simulink model "mimo_sim1"  (R2014a)
settings: Solver=ode45  StartTime=0.0  StopTime=20  RelTol=1e-3
values from neighbouring files (symbols this model uses):
  A = [A_lat, B_lat; zeros(2,5), [A_da 0; 0 A_dr]]    [session3.m]
  B = [zeros(5,2); B_da 0; 0 B_dr]    [session3.m]
  C = eye(7)    [session3.m]
  D = zeros(7,2)    [session3.m]
  k_phi = 0.1    [session3.m]
  k_psi = 2    [session3.m]
  k_r = 0.002    [session3.m]
settings Model: Creator=Bella Kim  LastModifiedBy=Bella Kim
settings DebuggingCC: SolverPrmCheckMsg=none

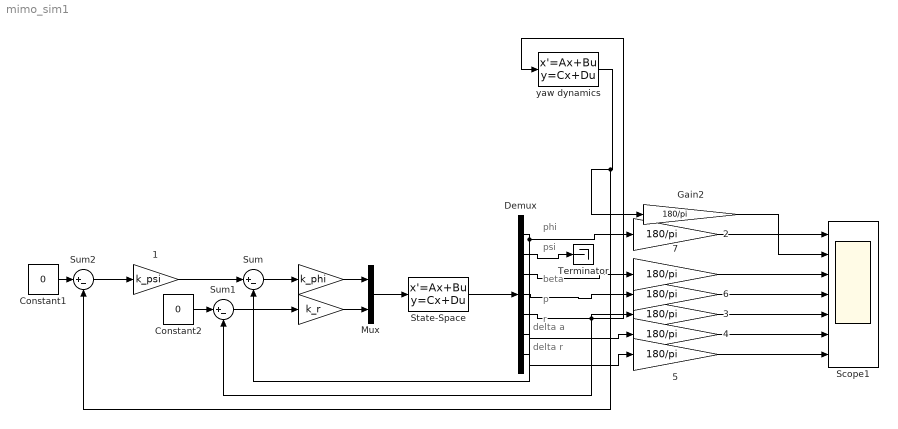
== system mimo_sim1 ==
  note: phi
  note: psi
  note: beta
  note: p
  note: r
  note: delta a
  note: delta r
  " " : Gain  Gain=k_r
  " " : Gain  Gain=k_phi
  " 1" : Gain  Gain=k_psi
   {2..7} (6 alike) : Gain  Gain=180/pi
  Constant1 : Constant  Value=0
  Constant2 : Constant  Value=0
  Demux : Demux  Outputs=7
  Gain2 : Gain  Gain=180/pi
  Mux : Mux  Inputs=2
  Scope1 : Scope  NumInputPorts=7
      settings: YMin=-5~-5~-5~-5~-5~-5~-5  YMax=5~5~5~5~5~5~5
  State-Space : StateSpace  A=A  B=B  C=C  D=D  X0=0
  Sum : Sum  Inputs=|+-
  Sum1 : Sum  Inputs=|+-
  Sum2 : Sum  Inputs=|+-
  Terminator : Terminator
  yaw dynamics : StateSpace  A=0  D=0  X0=30*pi/180
  wires:
  Mux/1 -> State-Space/1
  " "/1 -> Mux/1
  " "/1 -> Mux/2
  State-Space/1 -> Demux/1
  Demux/1 -> " 2"/1, Sum/2
  Sum/1 -> " "/1
  " 1"/1 -> Sum/1
  Constant2/1 -> Sum1/1
  Sum1/1 -> " "/1
  Sum2/1 -> " 1"/1
  Constant1/1 -> Sum2/1
  " 2"/1 -> Scope1/1
  " 5"/1 -> Scope1/7
  " 4"/1 -> Scope1/6
  " 3"/1 -> Scope1/5
  " 6"/1 -> Scope1/4
  " 7"/1 -> Scope1/3
  Demux/3 -> " 7"/1
  Demux/4 -> " 6"/1
  Demux/6 -> " 4"/1
  Demux/7 -> " 5"/1
  Demux/5 -> yaw dynamics/1, Sum1/2, " 3"/1
  Demux/2 -> Terminator/1
  Gain2/1 -> Scope1/2
  yaw dynamics/1 -> Gain2/1, Sum2/2
